simulink model "test_SOH_multi_cell"  (R2024a)
settings: Solver=FixedStepAuto  StartTime=0.0  StopTime=3600*24*365  FixedStep=1  RelTol=1e-3
libraries: simulink x1
settings Model: DataDictionary=SOXDictionaryGotion.sldd  Creator=mmackenzie  LastModifiedBy=mmackenzie
settings OptimizationCC: DefaultUnderspecifiedDataType=single
settings DebuggingCC: ParamPrecisionLossAbsoluteDiffThreshold=1e-10  ParamPrecisionLossRelativeDiffThreshold=1e-6  AllowSymbolicDim=off

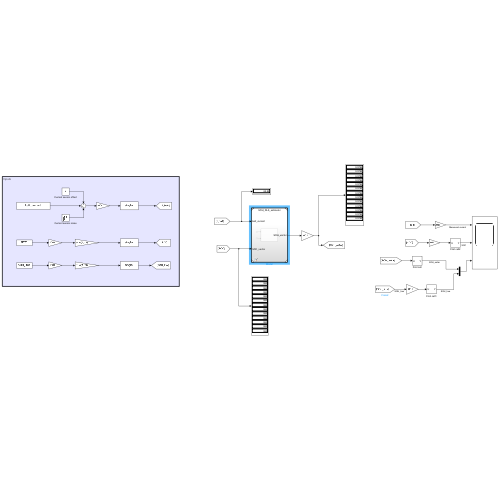
[thumbnail: Simulink's stored preview of the top-level diagram]
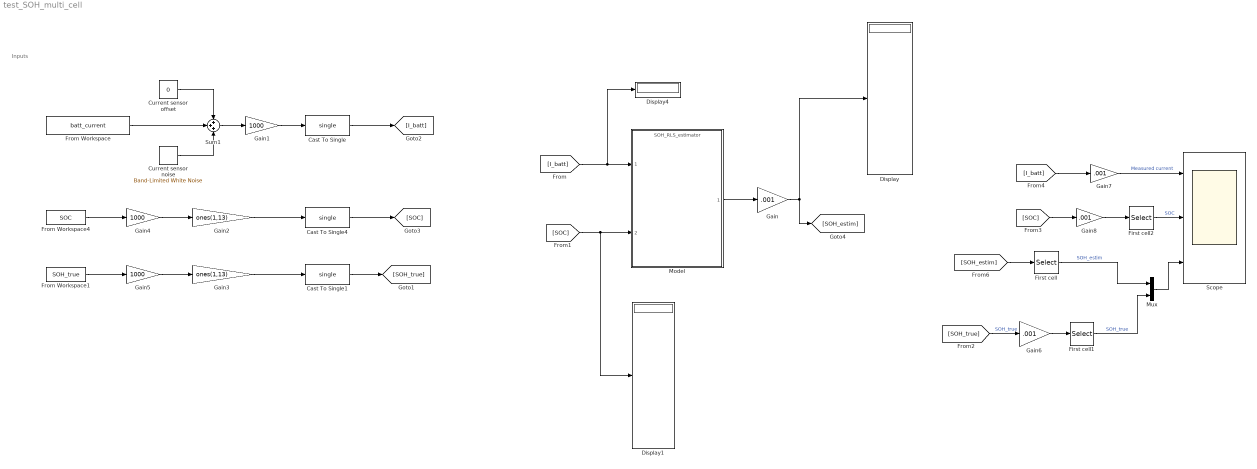
== system test_SOH_multi_cell ==
  note: Inputs
  Cast To Single : DataTypeConversion  OutDataTypeStr=single  SaturateOnIntegerOverflow=off  RndMeth=Floor
  Cast To Single1 : DataTypeConversion  OutDataTypeStr=single  SaturateOnIntegerOverflow=off  RndMeth=Floor
  Cast To Single4 : DataTypeConversion  OutDataTypeStr=single  SaturateOnIntegerOverflow=off  RndMeth=Floor
  Current sensor noise : simulink/Sources/Band-Limited White Noise  Cov=.1  Ts=1  seed=42
  Current sensor offset : Constant  Value=0
  Display : Display
  Display1 : Display
  Display4 : Display
  First cell : Selector  InputPortWidth=13  IndexOptions=Index vector (dialog)  Indices=1  OutputSizes=1
  First cell1 : Selector  InputPortWidth=13  IndexOptions=Index vector (dialog)  Indices=1  OutputSizes=1
  First cell2 : Selector  InputPortWidth=13  IndexOptions=Index vector (dialog)  Indices=1  OutputSizes=1
  From Workspace : FromWorkspace  VariableName=batt_current
  From Workspace1 : FromWorkspace  VariableName=SOH_true
  From Workspace4 : FromWorkspace  VariableName=SOC
  Gain{,6..8} (4 alike) : Gain  Gain=.001
  Gain1 : Gain  Gain=1000
  Gain2 : Gain  Gain=ones(1,13)
  Gain3 : Gain  Gain=ones(1,13)
  Gain4 : Gain  Gain=1000
  Gain5 : Gain  Gain=1000
  Model : ModelReference  ModelNameDialog=SOH_RLS_estimator.slx  SimulationMode=Normal  ModelReferenceVersion=1.42
  Mux : Mux  Inputs=2
  Scope : Scope  NumInputPorts=3
  Sum1 : Sum  Inputs=+++
  wires:
  [I_batt] -> Gain7/1
  Model/1 -> Gain/1
  [SOH_estim] -> First cell/1
  From Workspace/1 -> Sum1/2
  Current sensor offset/1 -> Sum1/1
  From Workspace4/1 -> Gain4/1
  Sum1/1 -> Gain1/1
  Current sensor noise/1 -> Sum1/3
  Gain/1 -> [SOH_estim], Display/1
  Gain1/1 -> Cast To Single/1
  Gain4/1 -> Gain2/1
  Cast To Single/1 -> [I_batt]
  Cast To Single4/1 -> [SOC]
  [I_batt] -> Display4/1, Model/1
  [SOC] -> Display1/1, Model/2
  Gain2/1 -> Cast To Single4/1
  Gain3/1 -> Cast To Single1/1
  Cast To Single1/1 -> [SOH_true]
  Gain5/1 -> Gain3/1
  From Workspace1/1 -> Gain5/1
  [SOH_true] -> Gain6/1  "SOH_true"
  Mux/1 -> Scope/3
  Gain6/1 -> First cell1/1
  [SOC] -> Gain8/1
  Gain7/1 -> Scope/1  "Measured current"
  Gain8/1 -> First cell2/1
  First cell/1 -> Mux/1  "SOH_estim"
  First cell1/1 -> Mux/2  "SOH_true"
  First cell2/1 -> Scope/2  "SOC"
